simulink library "lib_decmp_Calib_tbm_brkPreTriger_x6"  (R2020a)
settings: Solver=VariableStepAuto  StartTime=0.0  StopTime=10.0  RelTol=1e-3
settings Model: Creator=Administrator  LastModifiedBy=Administrator

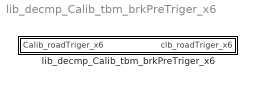
== system lib_decmp_Calib_tbm_brkPreTriger_x6 ==
  lib_decmp_Calib_tbm_brkPreTriger_x6 : Subsystem

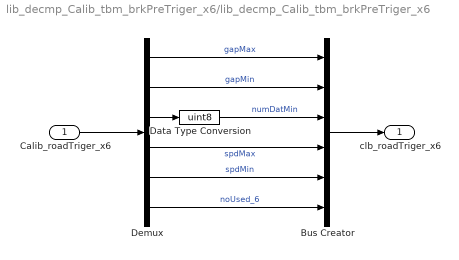
== system lib_decmp_Calib_tbm_brkPreTriger_x6/lib_decmp_Calib_tbm_brkPreTriger_x6 ==
  Calib_roadTriger_x6 : Inport  OutDataTypeStr=single  PortDimensions=6
  Bus Creator : BusCreator  Inputs=6
  Data Type Conversion : DataTypeConversion  OutDataTypeStr=uint8  RndMeth=Nearest
  Demux : Demux  Outputs=6
  clb_roadTriger_x6 : Outport  PortDimensions=6
  wires:
  Calib_roadTriger_x6/1 -> Demux/1
  Demux/1 -> Bus Creator/1  "gapMax"
  Demux/3 -> Data Type Conversion/1
  Demux/6 -> Bus Creator/6  "noUsed_6"
  Bus Creator/1 -> clb_roadTriger_x6/1
  Demux/2 -> Bus Creator/2  "gapMin"
  Data Type Conversion/1 -> Bus Creator/3  "numDatMin"
  Demux/4 -> Bus Creator/4  "spdMax"
  Demux/5 -> Bus Creator/5  "spdMin"
